simulink model "crazyflie_pid"  (R2019a)
settings: Solver=FixedStepAuto  StartTime=0.0  StopTime=40  FixedStep=0.002  MaxStep=0.01  RelTol=1e-4  EnableMultiTasking=on
values from neighbouring files (symbols this model uses):
  f_co_a0 = 5.484560e-4    (= 0.000548456)    [init.m]
  f_co_a1 = 1.032633e-6    (= 1.032633e-06)    [init.m]
  f_co_a2 = 2.130295e-11    [init.m]
  g = 9.8    [init.m]
  Ixx = 16.823890e-6    (= 1.682389e-05)    [init.m]
  Iyy = 16.823890e-6    (= 1.682389e-05)    [init.m]
  Izz = 29.808912e-6    (= 2.9808912e-05)    [init.m]
  L = 4.6e-3    (= 0.0046)    [init.m]
  m = 27e-3    (= 0.027)    [init.m]
  pid_PITCH_iLimit = 20    [init.m]
  pid_PITCH_kd = 0    [init.m]
  pid_PITCH_ki = 3    [init.m]
  pid_PITCH_kp = 6    [init.m]
  pid_PITCH_oLimit = 65535    [init.m]
  pid_PITCHRATE_iLimit = 33.3    [init.m]
  pid_PITCHRATE_kd = 2.5    [init.m]
  pid_PITCHRATE_ki = 500    [init.m]
  pid_PITCHRATE_kp = 250    [init.m]
  pid_PITCHRATE_oLimit = 65535    [init.m]
  pid_ROLL_iLimit = 20    [init.m]
  pid_ROLL_kd = 0    [init.m]
  pid_ROLL_ki = 3    [init.m]
  pid_ROLL_kp = 6    [init.m]
  pid_ROLL_oLimit = 65535    [init.m]
  pid_ROLLRATE_iLimit = 33.3    [init.m]
  pid_ROLLRATE_kd = 2.5    [init.m]
  pid_ROLLRATE_ki = 500    [init.m]
  pid_ROLLRATE_kp = 250    [init.m]
  pid_YAW_iLimit = 360    [init.m]
  pid_YAW_kd = 0.35    [init.m]
  pid_YAW_ki = 1    [init.m]
  pid_YAW_kp = 6    [init.m]
  pid_YAW_oLimit = 65535    [init.m]
  pid_YAWRATE_iLimit = 166.7    [init.m]
  pid_YAWRATE_kd = 0    [init.m]
  pid_YAWRATE_ki = 16.7    [init.m]
  pid_YAWRATE_kp = 120    [init.m]
  pid_YAWRATE_oLimit = 65535    [init.m]
  pidVX_iLimit = 5000    [init.m]
  pidVX_kd = 0    [init.m]
  pidVX_ki = 1    [init.m]
  pidVX_kp = 25    [init.m]
  pidVX_oLimit = rpLimit*overhead    (= 22)    [init.m]
  pidVY_iLimit = 5000    [init.m]
  pidVY_kd = 0    [init.m]
  pidVY_ki = 1    [init.m]
  pidVY_kp = 25    [init.m]
  pidVY_oLimit = rpLimit*overhead    (= 22)    [init.m]
  pidVZ_iLimit = 5000    [init.m]
  pidVZ_kd = 0    [init.m]
  pidVZ_ki = 15    [init.m]
  pidVZ_kp = 25    [init.m]
  pidVZ_oLimit = (65535/2/thrustScale)    (= 32.7675)    [init.m]
  pidX_iLimit = 5000    [init.m]
  pidX_kd = 0    [init.m]
  pidX_ki = 0    [init.m]
  pidX_kp = 1    [init.m]
  pidX_oLimit = velxmax*overhead    (= 1.1)    [init.m]
  pidY_iLimit = 5000    [init.m]
  pidY_kd = 0    [init.m]
  pidY_ki = 0    [init.m]
  pidY_kp = 1    [init.m]
  pidY_oLimit = velymax*overhead    (= 1.1)    [init.m]
  pidZ_iLimit = 5000    [init.m]
  pidZ_kd = 0    [init.m]
  pidZ_ki = 0.5    [init.m]
  pidZ_kp = 2    [init.m]
  pidZ_oLimit = min(velzmax,0.5)*overhead    [init.m]
  rpLimit = 20    [init.m]
  tau_co_a0 = 1.563383e-5    (= 1.563383e-05)    [init.m]
  tau_co_a1 = 0.005964552    [init.m]
  thrustBase = 36000    [init.m]
  thrustMin = 20000    [init.m]
  thrustScale = 1000    [init.m]
  yawd = 0    [init.m]    (also in trajectory.m)
undefined symbols (not defined in the file or in its folder): DiscIntNeverNeededParam
libraries: simulink x12, shared6dof x1
settings Model: Creator=Lucas  LastModifiedBy=Lucas
settings SolverCC: AutoInsertRateTranBlk=on
settings DataIOCC: LimitDataPoints=on  SaveOutput=off  SaveTime=off  ReturnWorkspaceOutputs=off
settings OptimizationCC: ExpressionDepthLimit=2147483647  LifeSpan=1
settings DebuggingCC: UnderspecifiedInitializationDetection=Classic  MergeDetectMultiDrivingBlocksExec=none  FcnCallInpInsideContextMsg=warning  AllowSymbolicDim=off  StateNameClashWarn=warning  SFUnexpectedBacktrackingDiag=warning  SFNoUnconditionalDefaultTransitionDiag=warning  SFExecutionAtInitializationDiag=none  ArithmeticOperatorsInVariantConditions=warning
settings SFSimCC: SimUseLocalCustomCode=off
settings RTWCC: RTWUseLocalCustomCode=off
settings CodeAppCC: StateflowObjectComments=on
settings GRTTargetCC: TargetLangStandard=C89/C90 (ANSI)  GeneratePreprocessorConditionals=Disable all  CombineOutputUpdateFcns=off  GRTInterface=on

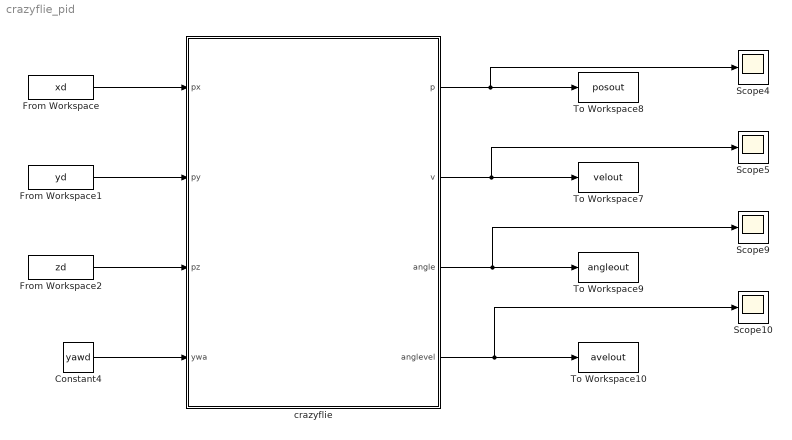
== system crazyflie_pid ==
  Constant4 : Constant  Value=yawd
  From Workspace : FromWorkspace  VariableName=xd  SampleTime=0
  From Workspace1 : FromWorkspace  VariableName=yd  SampleTime=0
  From Workspace2 : FromWorkspace  VariableName=zd  SampleTime=0
  Scope{4..5,9..10} (4 alike) : Scope
  To Workspace10 : ToWorkspace  VariableName=avelout  SaveFormat=Timeseries  SampleTime=-1
  To Workspace7 : ToWorkspace  VariableName=velout  SaveFormat=Timeseries  SampleTime=-1
  To Workspace8 : ToWorkspace  VariableName=posout  SaveFormat=Timeseries  SampleTime=-1
  To Workspace9 : ToWorkspace  VariableName=angleout  SaveFormat=Timeseries  SampleTime=-1
  crazyflie : Subsystem
  wires:
  crazyflie/1(p) -> Scope4/1, To Workspace8/1
  crazyflie/2(v) -> Scope5/1, To Workspace7/1
  crazyflie/3(angle) -> Scope9/1, To Workspace9/1
  crazyflie/4(anglevel) -> Scope10/1, To Workspace10/1
  Constant4/1 -> crazyflie/4(ywa)
  From Workspace/1 -> crazyflie/1(px)
  From Workspace1/1 -> crazyflie/2(py)
  From Workspace2/1 -> crazyflie/3(pz)

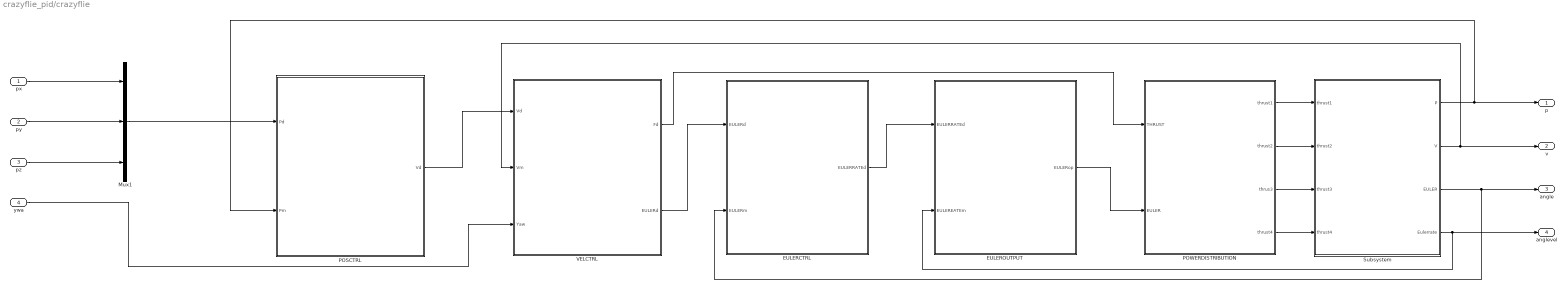
== system crazyflie_pid/crazyflie ==
  px : Inport
  py : Inport  Port=2
  pz : Inport  Port=3
  ywa : Inport  Port=4
  EULERCTRL : Subsystem  TreatAsAtomicUnit=on  SystemSampleTime=1/500
  EULEROUTPUT : Subsystem  TreatAsAtomicUnit=on  SystemSampleTime=1/500
  Mux1 : Mux  Inputs=3
  POSCTRL : Subsystem  TreatAsAtomicUnit=on  SystemSampleTime=1/100
      settings: AttributesFormatString=%<SystemSampleTime>=[10 0]
  POWERDISTRIBUTION : Subsystem  TreatAsAtomicUnit=on  SystemSampleTime=1/500
  Subsystem : Subsystem
  VELCTRL : Subsystem  TreatAsAtomicUnit=on  SystemSampleTime=1/100
  p : Outport
  v : Outport  Port=2
  angle : Outport  Port=3
  anglevel : Outport  Port=4
  wires:
  POWERDISTRIBUTION/2(thrust2) -> Subsystem/2(thrust2)
  Subsystem/2(V) -> v/1, VELCTRL/2(Vm)
  VELCTRL/2(EULERd) -> EULERCTRL/1(EULERd)
  POSCTRL/1(Vd) -> VELCTRL/1(Vd)
  Subsystem/3(EULER) -> angle/1, EULERCTRL/2(EULERm)
  POWERDISTRIBUTION/1(thrust1) -> Subsystem/1(thrust1)
  VELCTRL/1(Fd) -> POWERDISTRIBUTION/1(THRUST)
  Subsystem/1(P) -> POSCTRL/2(Pm), p/1
  POWERDISTRIBUTION/4(thrust4) -> Subsystem/4(thrust4)
  EULEROUTPUT/1(EULERop) -> POWERDISTRIBUTION/2(EULER)
  Subsystem/4(Eulerrate) -> anglevel/1, EULEROUTPUT/2(EULEREATEm)
  POWERDISTRIBUTION/3(thrus3) -> Subsystem/3(thrust3)
  EULERCTRL/1(EULERRATEd) -> EULEROUTPUT/1(EULERRATEd)
  pz/1 -> Mux1/3
  px/1 -> Mux1/1
  Mux1/1 -> POSCTRL/1(Pd)
  py/1 -> Mux1/2
  ywa/1 -> VELCTRL/3(Yaw)

== system crazyflie_pid/crazyflie/EULERCTRL ==
  EULERd : Inport
  EULERm : Inport  Port=2
  Add : Sum  Inputs=+|-
  Demux : Demux  Outputs=3
  Mux1 : Mux  Inputs=3
  PID1 : Subsystem
  PID2 : Subsystem
  PID3 : Subsystem
  EULERRATEd : Outport
  wires:
  PID2/1(PITCHRATEd) -> Mux1/2
  Demux/2 -> PID2/1(dPITCH)
  EULERd/1 -> Add/1
  Demux/1 -> PID1/1(dROLL)
  Add/1 -> Demux/1
  Demux/3 -> PID3/1(dYAW)
  PID3/1(YAWRATEd) -> Mux1/3
  EULERm/1 -> Add/2
  PID1/1(ROLLRATEd) -> Mux1/1
  Mux1/1 -> EULERRATEd/1

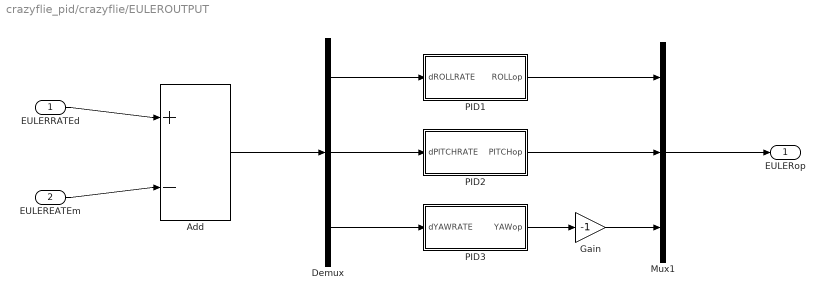
== system crazyflie_pid/crazyflie/EULEROUTPUT ==
  EULERRATEd : Inport
  EULEREATEm : Inport  Port=2
  Add : Sum  Inputs=+|-
  Demux : Demux  Outputs=3
  Gain : Gain  Gain=-1
  Mux1 : Mux  Inputs=3
  PID1 : Subsystem
  PID2 : Subsystem
  PID3 : Subsystem
  EULERop : Outport
  wires:
  PID2/1(PITCHop) -> Mux1/2
  Demux/2 -> PID2/1(dPITCHRATE)
  EULERRATEd/1 -> Add/1
  Demux/1 -> PID1/1(dROLLRATE)
  Add/1 -> Demux/1
  Demux/3 -> PID3/1(dYAWRATE)
  PID3/1(YAWop) -> Gain/1
  EULEREATEm/1 -> Add/2
  PID1/1(ROLLop) -> Mux1/1
  Mux1/1 -> EULERop/1
  Gain/1 -> Mux1/3

== system crazyflie_pid/crazyflie/POSCTRL ==
  Pd : Inport
  Pm : Inport  Port=2
  Add : Sum  Inputs=+|-
  Demux : Demux  Outputs=3
  Mux1 : Mux  Inputs=3
  PID1 : Subsystem
  PID2 : Subsystem
  PID3 : Subsystem
  Vd : Outport
  wires:
  Mux1/1 -> Vd/1
  Add/1 -> Demux/1
  Pd/1 -> Add/1
  Demux/1 -> PID1/1(dX)
  Demux/2 -> PID2/1(dY)
  PID1/1(VXd) -> Mux1/1
  PID2/1(VYd) -> Mux1/2
  PID3/1(VZd) -> Mux1/3
  Demux/3 -> PID3/1(dZ)
  Pm/1 -> Add/2

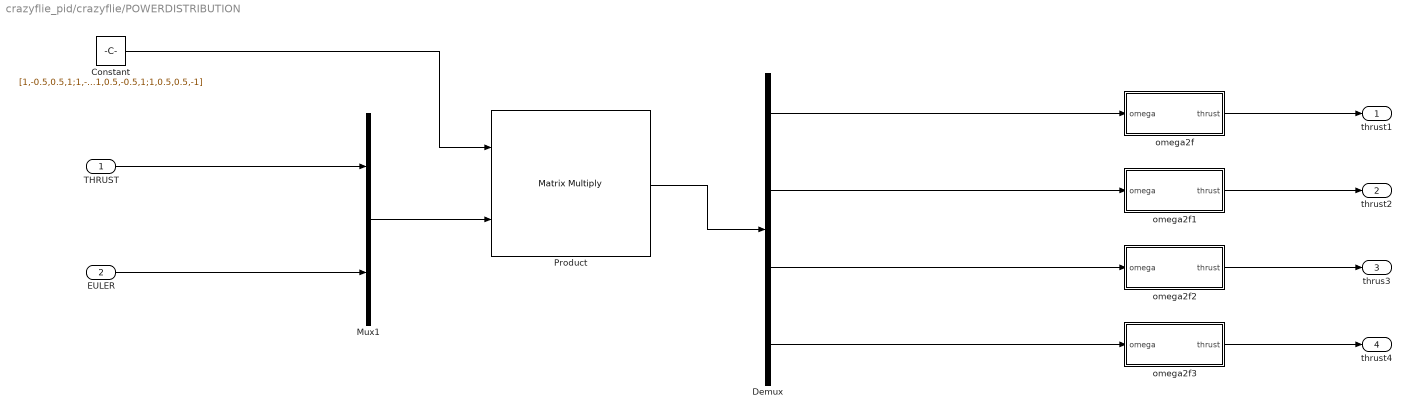
== system crazyflie_pid/crazyflie/POWERDISTRIBUTION ==
  THRUST : Inport
  EULER : Inport  Port=2
  Constant : Constant  Value=[1,-0.5,0.5,1;1,-0.5,-0.5,-1;1,0.5,-0.5,1;1,0.5,0.5,-1]
  Demux : Demux
  Mux1 : Mux  Inputs=2
  Product : Product  Multiplication=Matrix(*)
  omega2f : Subsystem
  omega2f1 : Subsystem
  omega2f2 : Subsystem
  omega2f3 : Subsystem
  thrust1 : Outport
  thrust2 : Outport  Port=2
  thrus3 : Outport  Port=3
  thrust4 : Outport  Port=4
  wires:
  EULER/1 -> Mux1/2
  THRUST/1 -> Mux1/1
  Mux1/1 -> Product/2
  Constant/1 -> Product/1
  Product/1 -> Demux/1
  Demux/1 -> omega2f/1(omega)
  Demux/2 -> omega2f1/1(omega)
  Demux/3 -> omega2f2/1(omega)
  Demux/4 -> omega2f3/1(omega)
  omega2f/1(thrust) -> thrust1/1
  omega2f1/1(thrust) -> thrust2/1
  omega2f2/1(thrust) -> thrus3/1
  omega2f3/1(thrust) -> thrust4/1

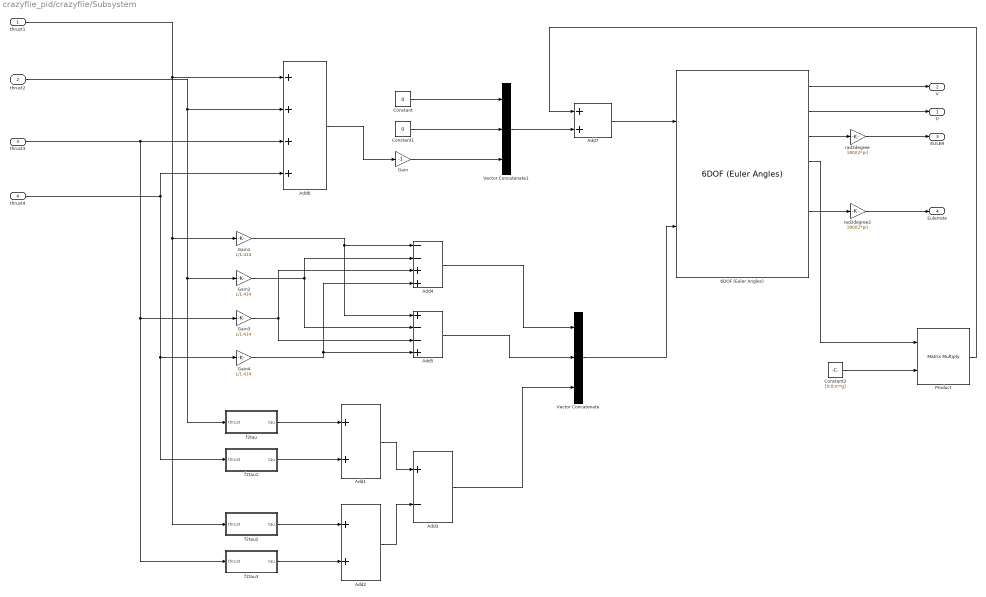
== system crazyflie_pid/crazyflie/Subsystem ==
  thrust1 : Inport
  thrust2 : Inport  Port=2
  thrust3 : Inport  Port=3
  thrust4 : Inport  Port=4
  6DOF (Euler Angles) : shared6dof/6DOF (Euler Angles)  units=Metric (MKS)  mtype=Fixed  rep=Euler Angles  xme_0=[0 0 0]  Vm_0=[0 0 0]  eul_0=[0 0 0]  pm_0=[0 0 0]  mass_0=m  mass_e=0.5  mass_f=2.0  inertia=[Ixx,0,0;0,Iyy,0;0,0,Izz]  inertia_e=eye(3)  inertia_f=2*eye(3)  k_quat=1.0  vre_flag=on  abi_flag=off  aMode=0  xme_statename=''  Vm_statename=''  eul_statename=''  quat_statename=''  pm_statename=''  mass_statename=''
      settings: SourceProductBaseCode=AE
  Add1 : Sum
  Add2 : Sum
  Add3 : Sum  Inputs=+-
  Add4 : Sum  Inputs=--++
  Add5 : Sum  Inputs=+--+
  Add6 : Sum  Inputs=++++
  Add7 : Sum
  Constant : Constant  Value=0
  Constant1 : Constant  Value=0
  Constant2 : Constant  Value=[0;0;m*g]
  Gain : Gain  Gain=-1
  Gain{1..4} (4 alike) : Gain  Gain=L/1.414
  Product : Product  Multiplication=Matrix(*)
  Vector Concatenate : Concatenate  NumInputs=3
  Vector Concatenate1 : Concatenate  NumInputs=3
  f2tau : Subsystem
  f2tau1 : Subsystem
  f2tau2 : Subsystem
  f2tau3 : Subsystem
  rad2degree : Gain  Gain=180/(2*pi)
  rad2degree2 : Gain  Gain=180/(2*pi)
  P : Outport
  V : Outport  Port=2
  EULER : Outport  Port=3
  Eulerrate : Outport  Port=4
  wires:
  f2tau/1(tau) -> Add1/1
  f2tau1/1(tau) -> Add1/2
  f2tau2/1(tau) -> Add2/1
  Add1/1 -> Add3/1
  Add2/1 -> Add3/2
  Add3/1 -> Vector Concatenate/3
  Constant/1 -> Vector Concatenate1/1
  Constant1/1 -> Vector Concatenate1/2
  Vector Concatenate/1 -> 6DOF (Euler Angles)/2
  6DOF (Euler Angles)/1 -> V/1
  6DOF (Euler Angles)/2 -> P/1
  Add7/1 -> 6DOF (Euler Angles)/1
  Product/1 -> Add7/1
  Vector Concatenate1/1 -> Add7/2
  Add6/1 -> Gain/1
  Gain/1 -> Vector Concatenate1/3
  6DOF (Euler Angles)/3 -> rad2degree/1
  rad2degree/1 -> EULER/1
  6DOF (Euler Angles)/6 -> rad2degree2/1
  rad2degree2/1 -> Eulerrate/1
  f2tau3/1(tau) -> Add2/2
  Gain1/1 -> Add5/1, Add4/1
  Gain3/1 -> Add5/3, Add4/3
  Gain4/1 -> Add4/4, Add5/4
  Gain2/1 -> Add5/2, Add4/2
  Add4/1 -> Vector Concatenate/1
  Add5/1 -> Vector Concatenate/2
  6DOF (Euler Angles)/4 -> Product/1
  Constant2/1 -> Product/2
  thrust1/1 -> f2tau2/1(thrust), Gain1/1, Add6/1
  thrust2/1 -> f2tau/1(thrust), Gain2/1, Add6/2
  thrust3/1 -> f2tau3/1(thrust), Gain3/1, Add6/3
  thrust4/1 -> f2tau1/1(thrust), Gain4/1, Add6/4

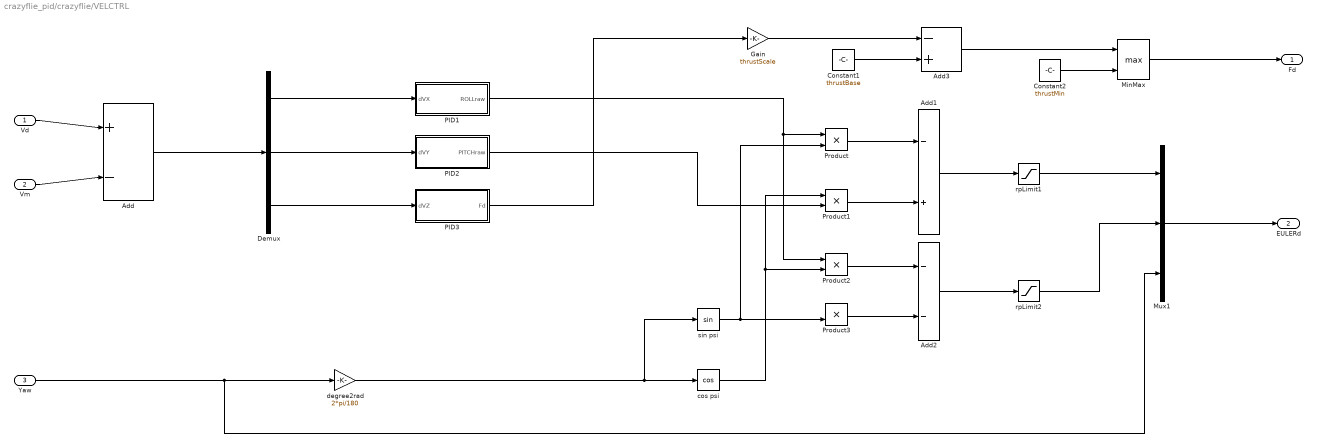
== system crazyflie_pid/crazyflie/VELCTRL ==
  Vd : Inport
  Vm : Inport  Port=2
  Yaw : Inport  Port=3
  Add : Sum  Inputs=+|-
  Add1 : Sum  Inputs=-+
  Add2 : Sum  Inputs=--
  Add3 : Sum  Inputs=-+
  Constant1 : Constant  Value=thrustBase
  Constant2 : Constant  Value=thrustMin
  Demux : Demux  Outputs=3
  Gain : Gain  Gain=thrustScale
  MinMax : MinMax  Function=max  Inputs=2
  Mux1 : Mux  Inputs=3
  PID1 : Subsystem
  PID2 : Subsystem
  PID3 : Subsystem
  Product{,1..3} (4 alike) : Product  RndMeth=Zero
  cos psi : Trigonometry  Operator=cos
  degree2rad : Gain  Gain=2*pi/180
  rpLimit1 : Saturate  UpperLimit=rpLimit  LowerLimit=-rpLimit
  rpLimit2 : Saturate  UpperLimit=rpLimit  LowerLimit=-rpLimit
  sin psi : Trigonometry
  Fd : Outport
  EULERd : Outport  Port=2
  wires:
  Demux/2 -> PID2/1(dVY)
  Vd/1 -> Add/1
  Demux/1 -> PID1/1(dVX)
  Add/1 -> Demux/1
  Demux/3 -> PID3/1(dVZ)
  PID3/1(Fd) -> Gain/1
  sin psi/1 -> Product/2, Product3/2
  PID2/1(PITCHraw) -> Product1/2
  PID1/1(ROLLraw) -> Product2/1, Product/1
  Product3/1 -> Add2/2
  Yaw/1 -> Mux1/3, degree2rad/1
  Product/1 -> Add1/1
  Product1/1 -> Add1/2
  cos psi/1 -> Product1/1, Product2/2
  Product2/1 -> Add2/1
  Add1/1 -> rpLimit1/1
  rpLimit1/1 -> Mux1/1
  Add2/1 -> rpLimit2/1
  rpLimit2/1 -> Mux1/2
  Mux1/1 -> EULERd/1
  Constant1/1 -> Add3/2
  Gain/1 -> Add3/1
  Add3/1 -> MinMax/1
  degree2rad/1 -> sin psi/1, cos psi/1
  Constant2/1 -> MinMax/2
  MinMax/1 -> Fd/1
  Vm/1 -> Add/2

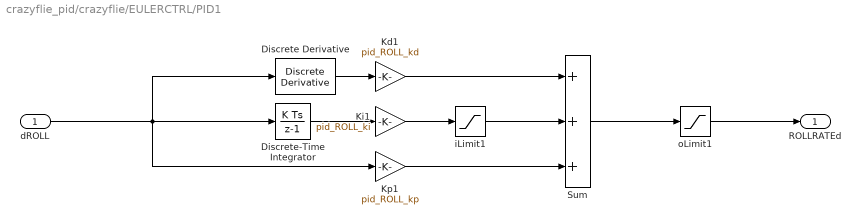
== system crazyflie_pid/crazyflie/EULERCTRL/PID1 ==
  dROLL : Inport
  Discrete Derivative : simulink/Discrete/Discrete Derivative  gainval=1.0  ICPrevScaledInput=0.0  OutMin=[]  OutMax=[]  OutDataType=fixdt(1, 16)  OutScaling=2^-10  DoSatur=off
  Discrete-Time Integrator : DiscreteIntegrator  SampleTime=-1  ICPrevOutput=DiscIntNeverNeededParam  ICPrevScaledInput=DiscIntNeverNeededParam
  Kd1 : Gain  Gain=pid_ROLL_kd
  Ki1 : Gain  Gain=pid_ROLL_ki
  Kp1 : Gain  Gain=pid_ROLL_kp
  Sum : Sum  Inputs=+++
  iLimit1 : Saturate  UpperLimit=pid_ROLL_iLimit  LowerLimit=-pid_ROLL_iLimit
  oLimit1 : Saturate  UpperLimit=pid_ROLL_oLimit  LowerLimit=-pid_ROLL_oLimit
  ROLLRATEd : Outport
  wires:
  Discrete-Time Integrator/1 -> Ki1/1
  iLimit1/1 -> Sum/2
  Kp1/1 -> Sum/3
  Kd1/1 -> Sum/1
  Sum/1 -> oLimit1/1
  Ki1/1 -> iLimit1/1
  Discrete Derivative/1 -> Kd1/1
  dROLL/1 -> Discrete-Time Integrator/1, Discrete Derivative/1, Kp1/1
  oLimit1/1 -> ROLLRATEd/1

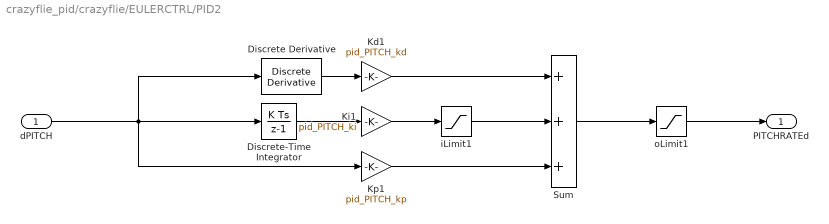
== system crazyflie_pid/crazyflie/EULERCTRL/PID2 ==
  dPITCH : Inport
  Discrete Derivative : simulink/Discrete/Discrete Derivative  gainval=1.0  ICPrevScaledInput=0.0  OutMin=[]  OutMax=[]  OutDataType=fixdt(1, 16)  OutScaling=2^-10  DoSatur=off
  Discrete-Time Integrator : DiscreteIntegrator  SampleTime=-1  ICPrevOutput=DiscIntNeverNeededParam  ICPrevScaledInput=DiscIntNeverNeededParam
  Kd1 : Gain  Gain=pid_PITCH_kd
  Ki1 : Gain  Gain=pid_PITCH_ki
  Kp1 : Gain  Gain=pid_PITCH_kp
  Sum : Sum  Inputs=+++
  iLimit1 : Saturate  UpperLimit=pid_PITCH_iLimit  LowerLimit=-pid_PITCH_iLimit
  oLimit1 : Saturate  UpperLimit=pid_PITCH_oLimit  LowerLimit=-pid_PITCH_oLimit
  PITCHRATEd : Outport
  wires:
  Discrete-Time Integrator/1 -> Ki1/1
  iLimit1/1 -> Sum/2
  Kp1/1 -> Sum/3
  Kd1/1 -> Sum/1
  Sum/1 -> oLimit1/1
  Ki1/1 -> iLimit1/1
  Discrete Derivative/1 -> Kd1/1
  dPITCH/1 -> Discrete Derivative/1, Discrete-Time Integrator/1, Kp1/1
  oLimit1/1 -> PITCHRATEd/1

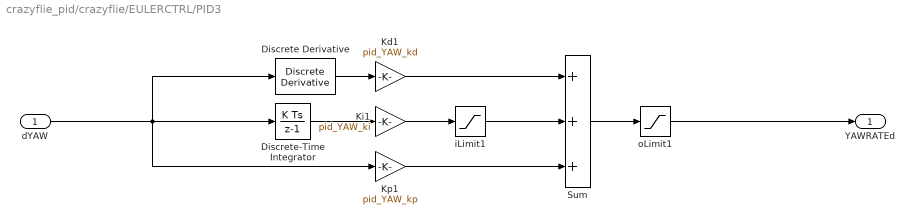
== system crazyflie_pid/crazyflie/EULERCTRL/PID3 ==
  dYAW : Inport
  Discrete Derivative : simulink/Discrete/Discrete Derivative  gainval=1.0  ICPrevScaledInput=0.0  OutMin=[]  OutMax=[]  OutDataType=fixdt(1, 16)  OutScaling=2^-10  DoSatur=off
  Discrete-Time Integrator : DiscreteIntegrator  SampleTime=-1  ICPrevOutput=DiscIntNeverNeededParam  ICPrevScaledInput=DiscIntNeverNeededParam
  Kd1 : Gain  Gain=pid_YAW_kd
  Ki1 : Gain  Gain=pid_YAW_ki
  Kp1 : Gain  Gain=pid_YAW_kp
  Sum : Sum  Inputs=+++
  iLimit1 : Saturate  UpperLimit=pid_YAW_iLimit  LowerLimit=-pid_YAW_iLimit
  oLimit1 : Saturate  UpperLimit=pid_YAW_oLimit  LowerLimit=-pid_YAW_oLimit
  YAWRATEd : Outport
  wires:
  Discrete-Time Integrator/1 -> Ki1/1
  iLimit1/1 -> Sum/2
  Kp1/1 -> Sum/3
  Kd1/1 -> Sum/1
  Sum/1 -> oLimit1/1
  Ki1/1 -> iLimit1/1
  Discrete Derivative/1 -> Kd1/1
  dYAW/1 -> Discrete-Time Integrator/1, Discrete Derivative/1, Kp1/1
  oLimit1/1 -> YAWRATEd/1

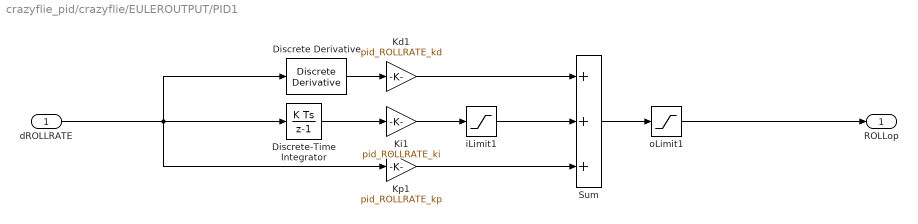
== system crazyflie_pid/crazyflie/EULEROUTPUT/PID1 ==
  dROLLRATE : Inport
  Discrete Derivative : simulink/Discrete/Discrete Derivative  gainval=1.0  ICPrevScaledInput=0.0  OutMin=[]  OutMax=[]  OutDataType=fixdt(1, 16)  OutScaling=2^-10  DoSatur=off
  Discrete-Time Integrator : DiscreteIntegrator  SampleTime=-1  ICPrevOutput=DiscIntNeverNeededParam  ICPrevScaledInput=DiscIntNeverNeededParam
  Kd1 : Gain  Gain=pid_ROLLRATE_kd
  Ki1 : Gain  Gain=pid_ROLLRATE_ki
  Kp1 : Gain  Gain=pid_ROLLRATE_kp
  Sum : Sum  Inputs=+++
  iLimit1 : Saturate  UpperLimit=pid_ROLLRATE_iLimit  LowerLimit=-pid_ROLLRATE_iLimit
  oLimit1 : Saturate  UpperLimit=pid_ROLL_oLimit  LowerLimit=-pid_ROLL_oLimit
  ROLLop : Outport
  wires:
  Discrete-Time Integrator/1 -> Ki1/1
  iLimit1/1 -> Sum/2
  Kp1/1 -> Sum/3
  Kd1/1 -> Sum/1
  Sum/1 -> oLimit1/1
  Ki1/1 -> iLimit1/1
  Discrete Derivative/1 -> Kd1/1
  dROLLRATE/1 -> Discrete Derivative/1, Discrete-Time Integrator/1, Kp1/1
  oLimit1/1 -> ROLLop/1

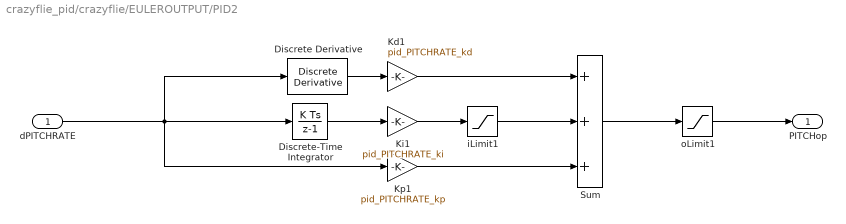
== system crazyflie_pid/crazyflie/EULEROUTPUT/PID2 ==
  dPITCHRATE : Inport
  Discrete Derivative : simulink/Discrete/Discrete Derivative  gainval=1.0  ICPrevScaledInput=0.0  OutMin=[]  OutMax=[]  OutDataType=fixdt(1, 16)  OutScaling=2^-10  DoSatur=off
  Discrete-Time Integrator : DiscreteIntegrator  SampleTime=-1  ICPrevOutput=DiscIntNeverNeededParam  ICPrevScaledInput=DiscIntNeverNeededParam
  Kd1 : Gain  Gain=pid_PITCHRATE_kd
  Ki1 : Gain  Gain=pid_PITCHRATE_ki
  Kp1 : Gain  Gain=pid_PITCHRATE_kp
  Sum : Sum  Inputs=+++
  iLimit1 : Saturate  UpperLimit=pid_PITCHRATE_iLimit  LowerLimit=-pid_PITCHRATE_iLimit
  oLimit1 : Saturate  UpperLimit=pid_PITCHRATE_oLimit  LowerLimit=-pid_PITCHRATE_oLimit
  PITCHop : Outport
  wires:
  iLimit1/1 -> Sum/2
  Kp1/1 -> Sum/3
  Kd1/1 -> Sum/1
  Sum/1 -> oLimit1/1
  Ki1/1 -> iLimit1/1
  dPITCHRATE/1 -> Discrete-Time Integrator/1, Discrete Derivative/1, Kp1/1
  oLimit1/1 -> PITCHop/1
  Discrete Derivative/1 -> Kd1/1
  Discrete-Time Integrator/1 -> Ki1/1

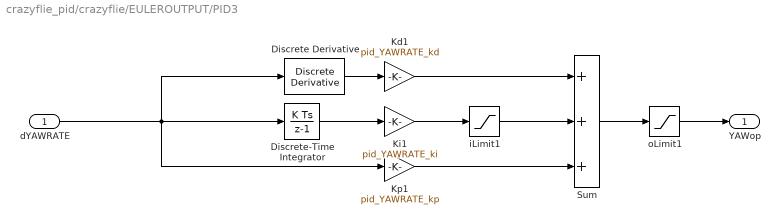
== system crazyflie_pid/crazyflie/EULEROUTPUT/PID3 ==
  dYAWRATE : Inport
  Discrete Derivative : simulink/Discrete/Discrete Derivative  gainval=1.0  ICPrevScaledInput=0.0  OutMin=[]  OutMax=[]  OutDataType=fixdt(1, 16)  OutScaling=2^-10  DoSatur=off
  Discrete-Time Integrator : DiscreteIntegrator  SampleTime=-1  ICPrevOutput=DiscIntNeverNeededParam  ICPrevScaledInput=DiscIntNeverNeededParam
  Kd1 : Gain  Gain=pid_YAWRATE_kd
  Ki1 : Gain  Gain=pid_YAWRATE_ki
  Kp1 : Gain  Gain=pid_YAWRATE_kp
  Sum : Sum  Inputs=+++
  iLimit1 : Saturate  UpperLimit=pid_YAWRATE_iLimit  LowerLimit=-pid_YAWRATE_iLimit
  oLimit1 : Saturate  UpperLimit=pid_YAWRATE_oLimit  LowerLimit=-pid_YAWRATE_oLimit
  YAWop : Outport
  wires:
  Discrete-Time Integrator/1 -> Ki1/1
  iLimit1/1 -> Sum/2
  Kp1/1 -> Sum/3
  Kd1/1 -> Sum/1
  Sum/1 -> oLimit1/1
  Ki1/1 -> iLimit1/1
  Discrete Derivative/1 -> Kd1/1
  dYAWRATE/1 -> Discrete Derivative/1, Discrete-Time Integrator/1, Kp1/1
  oLimit1/1 -> YAWop/1

== system crazyflie_pid/crazyflie/POSCTRL/PID1 ==
  dX : Inport
  Discrete Derivative : simulink/Discrete/Discrete Derivative  gainval=1  ICPrevScaledInput=0.0  OutMin=[]  OutMax=[]  OutDataType=fixdt(1, 16)  OutScaling=2^-10  DoSatur=off
  Discrete-Time Integrator : DiscreteIntegrator  SampleTime=-1  ICPrevOutput=DiscIntNeverNeededParam  ICPrevScaledInput=DiscIntNeverNeededParam
  Kd1 : Gain  Gain=pidX_kd
  Ki1 : Gain  Gain=pidX_ki
  Kp1 : Gain  Gain=pidX_kp
  Sum : Sum  Inputs=+++
  iLimit1 : Saturate  UpperLimit=pidX_iLimit  LowerLimit=-pidX_iLimit
  oLimit1 : Saturate  UpperLimit=pidX_oLimit  LowerLimit=-pidX_oLimit
  VXd : Outport
  wires:
  Discrete-Time Integrator/1 -> Ki1/1
  iLimit1/1 -> Sum/2
  Kp1/1 -> Sum/3
  Kd1/1 -> Sum/1
  Sum/1 -> oLimit1/1
  Ki1/1 -> iLimit1/1
  dX/1 -> Discrete Derivative/1, Discrete-Time Integrator/1, Kp1/1
  oLimit1/1 -> VXd/1
  Discrete Derivative/1 -> Kd1/1

== system crazyflie_pid/crazyflie/POSCTRL/PID2 ==
  dY : Inport
  Discrete Derivative : simulink/Discrete/Discrete Derivative  gainval=1.0  ICPrevScaledInput=0.0  OutMin=[]  OutMax=[]  OutDataType=fixdt(1, 16)  OutScaling=2^-10  DoSatur=off
  Discrete-Time Integrator : DiscreteIntegrator  SampleTime=-1  ICPrevOutput=DiscIntNeverNeededParam  ICPrevScaledInput=DiscIntNeverNeededParam
  Kd1 : Gain  Gain=pidY_kd
  Ki1 : Gain  Gain=pidY_ki
  Kp1 : Gain  Gain=pidY_kp
  Sum : Sum  Inputs=+++
  iLimit1 : Saturate  UpperLimit=pidY_iLimit  LowerLimit=-pidY_iLimit
  oLimit1 : Saturate  UpperLimit=pidY_oLimit  LowerLimit=-pidY_oLimit
  VYd : Outport
  wires:
  Discrete-Time Integrator/1 -> Ki1/1
  iLimit1/1 -> Sum/2
  Kp1/1 -> Sum/3
  Kd1/1 -> Sum/1
  Sum/1 -> oLimit1/1
  Ki1/1 -> iLimit1/1
  Discrete Derivative/1 -> Kd1/1
  dY/1 -> Discrete-Time Integrator/1, Discrete Derivative/1, Kp1/1
  oLimit1/1 -> VYd/1

== system crazyflie_pid/crazyflie/POSCTRL/PID3 ==
  dZ : Inport
  Discrete Derivative : simulink/Discrete/Discrete Derivative  gainval=1.0  ICPrevScaledInput=0.0  OutMin=[]  OutMax=[]  OutDataType=fixdt(1, 16)  OutScaling=2^-10  DoSatur=off
  Discrete-Time Integrator : DiscreteIntegrator  SampleTime=-1  ICPrevOutput=DiscIntNeverNeededParam  ICPrevScaledInput=DiscIntNeverNeededParam
  Kd1 : Gain  Gain=pidZ_kd
  Ki1 : Gain  Gain=pidZ_ki
  Kp1 : Gain  Gain=pidZ_kp
  Sum : Sum  Inputs=+++
  iLimit1 : Saturate  UpperLimit=pidZ_iLimit  LowerLimit=-pidZ_iLimit
  oLimit1 : Saturate  UpperLimit=pidZ_oLimit  LowerLimit=-pidZ_oLimit
  VZd : Outport
  wires:
  Discrete-Time Integrator/1 -> Ki1/1
  iLimit1/1 -> Sum/2
  Kp1/1 -> Sum/3
  Kd1/1 -> Sum/1
  Sum/1 -> oLimit1/1
  Ki1/1 -> iLimit1/1
  Discrete Derivative/1 -> Kd1/1
  dZ/1 -> Discrete Derivative/1, Discrete-Time Integrator/1, Kp1/1
  oLimit1/1 -> VZd/1

== system crazyflie_pid/crazyflie/POWERDISTRIBUTION/omega2f ==
  omega : Inport
  Add : Sum  Inputs=+++
  Constant : Constant  Value=f_co_a2
  Constant1 : Constant  Value=f_co_a1
  Constant2 : Constant  Value=f_co_a0
  Math Function : Math  Operator=square  SaturateOnIntegerOverflow=on
  Product : Product
  Product1 : Product
  thrust : Outport
  wires:
  omega/1 -> Product1/2, Math Function/1
  Constant/1 -> Product/1
  Math Function/1 -> Product/2
  Constant1/1 -> Product1/1
  Product/1 -> Add/1
  Product1/1 -> Add/2
  Constant2/1 -> Add/3
  Add/1 -> thrust/1

== system crazyflie_pid/crazyflie/POWERDISTRIBUTION/omega2f1 ==
  omega : Inport
  Add : Sum  Inputs=+++
  Constant : Constant  Value=f_co_a2
  Constant1 : Constant  Value=f_co_a1
  Constant2 : Constant  Value=f_co_a0
  Math Function : Math  Operator=square  SaturateOnIntegerOverflow=on
  Product : Product
  Product1 : Product
  thrust : Outport
  wires:
  omega/1 -> Product1/2, Math Function/1
  Constant/1 -> Product/1
  Math Function/1 -> Product/2
  Constant1/1 -> Product1/1
  Product/1 -> Add/1
  Product1/1 -> Add/2
  Constant2/1 -> Add/3
  Add/1 -> thrust/1

== system crazyflie_pid/crazyflie/POWERDISTRIBUTION/omega2f2 ==
  omega : Inport
  Add : Sum  Inputs=+++
  Constant : Constant  Value=f_co_a2
  Constant1 : Constant  Value=f_co_a1
  Constant2 : Constant  Value=f_co_a0
  Math Function : Math  Operator=square  SaturateOnIntegerOverflow=on
  Product : Product
  Product1 : Product
  thrust : Outport
  wires:
  omega/1 -> Product1/2, Math Function/1
  Constant/1 -> Product/1
  Math Function/1 -> Product/2
  Constant1/1 -> Product1/1
  Product/1 -> Add/1
  Product1/1 -> Add/2
  Constant2/1 -> Add/3
  Add/1 -> thrust/1

== system crazyflie_pid/crazyflie/POWERDISTRIBUTION/omega2f3 ==
  omega : Inport
  Add : Sum  Inputs=+++
  Constant : Constant  Value=f_co_a2
  Constant1 : Constant  Value=f_co_a1
  Constant2 : Constant  Value=f_co_a0
  Math Function : Math  Operator=square  SaturateOnIntegerOverflow=on
  Product : Product
  Product1 : Product
  thrust : Outport
  wires:
  omega/1 -> Product1/2, Math Function/1
  Constant/1 -> Product/1
  Math Function/1 -> Product/2
  Constant1/1 -> Product1/1
  Product/1 -> Add/1
  Product1/1 -> Add/2
  Constant2/1 -> Add/3
  Add/1 -> thrust/1

== system crazyflie_pid/crazyflie/Subsystem/f2tau ==
  thrust : Inport
  Add : Sum
  Constant : Constant  Value=tau_co_a1
  Constant1 : Constant  Value=tau_co_a0
  Product : Product
  tau : Outport
  wires:
  thrust/1 -> Product/1
  Constant/1 -> Product/2
  Constant1/1 -> Add/2
  Product/1 -> Add/1
  Add/1 -> tau/1

== system crazyflie_pid/crazyflie/Subsystem/f2tau1 ==
  thrust : Inport
  Add : Sum
  Constant : Constant  Value=tau_co_a1
  Constant1 : Constant  Value=tau_co_a0
  Product : Product
  tau : Outport
  wires:
  thrust/1 -> Product/1
  Constant/1 -> Product/2
  Constant1/1 -> Add/2
  Product/1 -> Add/1
  Add/1 -> tau/1

== system crazyflie_pid/crazyflie/Subsystem/f2tau2 ==
  thrust : Inport
  Add : Sum
  Constant : Constant  Value=tau_co_a1
  Constant1 : Constant  Value=tau_co_a0
  Product : Product
  tau : Outport
  wires:
  thrust/1 -> Product/1
  Constant/1 -> Product/2
  Constant1/1 -> Add/2
  Product/1 -> Add/1
  Add/1 -> tau/1

== system crazyflie_pid/crazyflie/Subsystem/f2tau3 ==
  thrust : Inport
  Add : Sum
  Constant : Constant  Value=tau_co_a1
  Constant1 : Constant  Value=tau_co_a0
  Product : Product
  tau : Outport
  wires:
  thrust/1 -> Product/1
  Constant/1 -> Product/2
  Constant1/1 -> Add/2
  Product/1 -> Add/1
  Add/1 -> tau/1

== system crazyflie_pid/crazyflie/VELCTRL/PID1 ==
  dVX : Inport
  Discrete Derivative : simulink/Discrete/Discrete Derivative  gainval=1.0  ICPrevScaledInput=0.0  OutMin=[]  OutMax=[]  OutDataType=fixdt(1, 16)  OutScaling=2^-10  DoSatur=off
  Discrete-Time Integrator : DiscreteIntegrator  SampleTime=-1  ICPrevOutput=DiscIntNeverNeededParam  ICPrevScaledInput=DiscIntNeverNeededParam
  Kd1 : Gain  Gain=pidVX_kd
  Ki1 : Gain  Gain=pidVX_ki
  Kp1 : Gain  Gain=pidVX_kp
  Sum : Sum  Inputs=+++
  iLimit1 : Saturate  UpperLimit=pidVX_iLimit  LowerLimit=-pidVX_iLimit
  oLimit1 : Saturate  UpperLimit=pidVX_oLimit  LowerLimit=-pidVX_oLimit
  ROLLraw : Outport
  wires:
  Discrete-Time Integrator/1 -> Ki1/1
  iLimit1/1 -> Sum/2
  Kp1/1 -> Sum/3
  Kd1/1 -> Sum/1
  Sum/1 -> oLimit1/1
  Ki1/1 -> iLimit1/1
  Discrete Derivative/1 -> Kd1/1
  dVX/1 -> Discrete-Time Integrator/1, Kp1/1, Discrete Derivative/1
  oLimit1/1 -> ROLLraw/1

== system crazyflie_pid/crazyflie/VELCTRL/PID2 ==
  dVY : Inport
  Discrete Derivative : simulink/Discrete/Discrete Derivative  gainval=1.0  ICPrevScaledInput=0.0  OutMin=[]  OutMax=[]  OutDataType=fixdt(1, 16)  OutScaling=2^-10  DoSatur=off
  Discrete-Time Integrator : DiscreteIntegrator  SampleTime=-1  ICPrevOutput=DiscIntNeverNeededParam  ICPrevScaledInput=DiscIntNeverNeededParam
  Kd1 : Gain  Gain=pidVY_kd
  Ki1 : Gain  Gain=pidVY_ki
  Kp1 : Gain  Gain=pidVY_kp
  Sum : Sum  Inputs=+++
  iLimit1 : Saturate  UpperLimit=pidVY_iLimit  LowerLimit=-pidVY_iLimit
  oLimit1 : Saturate  UpperLimit=pidVY_oLimit  LowerLimit=-pidVY_oLimit
  PITCHraw : Outport
  wires:
  Discrete-Time Integrator/1 -> Ki1/1
  iLimit1/1 -> Sum/2
  Kp1/1 -> Sum/3
  Kd1/1 -> Sum/1
  Sum/1 -> oLimit1/1
  Ki1/1 -> iLimit1/1
  Discrete Derivative/1 -> Kd1/1
  dVY/1 -> Discrete Derivative/1, Discrete-Time Integrator/1, Kp1/1
  oLimit1/1 -> PITCHraw/1

== system crazyflie_pid/crazyflie/VELCTRL/PID3 ==
  dVZ : Inport
  Discrete Derivative : simulink/Discrete/Discrete Derivative  gainval=1.0  ICPrevScaledInput=0.0  OutMin=[]  OutMax=[]  OutDataType=fixdt(1, 16)  OutScaling=2^-10  DoSatur=off
  Discrete-Time Integrator : DiscreteIntegrator  SampleTime=-1  ICPrevOutput=DiscIntNeverNeededParam  ICPrevScaledInput=DiscIntNeverNeededParam
  Kd1 : Gain  Gain=pidVZ_kd
  Ki1 : Gain  Gain=pidVZ_ki
  Kp1 : Gain  Gain=pidVZ_kp
  Sum : Sum  Inputs=+++
  iLimit1 : Saturate  UpperLimit=pidVZ_iLimit  LowerLimit=-pidVZ_iLimit
  oLimit1 : Saturate  UpperLimit=pidVZ_oLimit  LowerLimit=-pidVZ_oLimit
  Fd : Outport
  wires:
  iLimit1/1 -> Sum/2
  Kp1/1 -> Sum/3
  Kd1/1 -> Sum/1
  Sum/1 -> oLimit1/1
  Ki1/1 -> iLimit1/1
  dVZ/1 -> Discrete-Time Integrator/1, Kp1/1, Discrete Derivative/1
  oLimit1/1 -> Fd/1
  Discrete Derivative/1 -> Kd1/1
  Discrete-Time Integrator/1 -> Ki1/1
